simulink model "BoostConverterTestEnviroment"  (R2020a)
settings: Solver=ode15s  StartTime=0.0  StopTime=0.05  RelTol=1e-3
libraries: ee_lib x2, fl_lib x1, nesl_utility x1
settings Model: Creator=ykamatan  LastModifiedBy=ykamatan
settings SolverCC: MaxConsecutiveMinStep=10
settings DataIOCC: SaveOutput=off  SaveTime=off

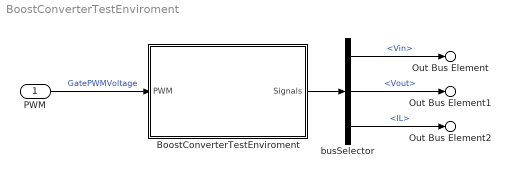
== system BoostConverterTestEnviroment ==
  PWM : Inport  OutDataTypeStr=double  PortDimensions=1  SampleTime=[2e-08,0]
  BoostConverterTestEnviroment : Subsystem  TreatAsAtomicUnit=on
  busSelector : BusSelector  OutputSignals=Vin,Vout,IL
  Out Bus Element : Outport  PortName=Signals  Element=Vin
  Out Bus Element1 : Outport  PortName=Signals  Element=Vout
  Out Bus Element2 : Outport  PortName=Signals  Element=IL
  wires:
  busSelector/3 -> Out Bus Element2/1  "<IL>"
  busSelector/2 -> Out Bus Element1/1  "<Vout>"
  busSelector/1 -> Out Bus Element/1  "<Vin>"
  BoostConverterTestEnviroment/1(Signals) -> busSelector/1
  PWM/1 -> BoostConverterTestEnviroment/1(PWM)  "GatePWMVoltage"

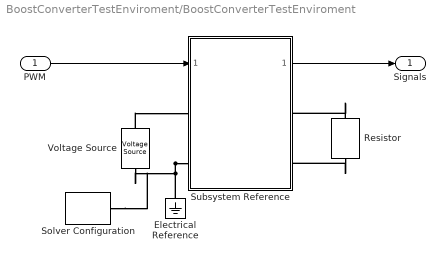
== system BoostConverterTestEnviroment/BoostConverterTestEnviroment ==
  PWM : Inport
  Electrical Reference : fl_lib/Electrical/Electrical Elements/Electrical Reference
  Resistor : ee_lib/Passive/Resistor  R=40 Ohm  R_tol=5  enable_R_tol=0  tol_distribution=1  nSigma=4  enable_operating_limits=0  operating_limit_action=2  max_working_voltage=100 V  power_rating=1 W  enable_faults=0  fault_action=1  R_faulted=inf Ohm  enable_temporal_fault=0  t_fault=1 s  enable_behavioral_fault=0  max_permissible_current=1 A  t_fail_on_current=1 s  noise_mode=0  sample_time=1e-3 s  repeatability=1  auto_seed=4144164703  user_seed=0  Tdevice=25 degC  alpha=3.93e-3 1/K  Tmeas=25 degC  thermal_mass=100 J/K  power_derating_T1=70 degC  power_derating_T2=155 degC  operating_temperature_range_vec=[-50, 150] degC  temperature_specify=off  temperature_priority=High  temperature=298.15 K  temperature_nominal_specify=off  temperature_nominal_unit=K  temperature_nominal_value=1
  Solver Configuration : nesl_utility/Solver Configuration  PhysicalDomain=network_engine_domain  SubClassName=solver  LeftPortType=input  RightPortType=generic  Tones=[]  Harmonics=[]  SimulateNoise=off  Profile=off  UseLocalSampling=off  EnableSwitchedLinearOptims=on  FrequencyDomain=off  UseCCode=off  RelTol=0.001  AbsTol=1e-06  MinStep=1e-09  ToWorkspace=off  RevertToSquareIcSolve=off  NumHomotopyIterations=100  PhasorMode=off  PhasorModeNumHarmonics=1  DoDC=off  ResidualTolerance=1e-09  UseLocalSolver=off  LocalSolverChoice=NE_BACKWARD_EULER_ADVANCER  LocalSolverSampleTime=0.001  DoFixedCost=off  MaxNonlinIter=3  MaxModeIter=2  LinearAlgebra=auto  EquationFormulation=NE_TIME_EF  DelaysMemoryBudget=1024  AutomaticFiltering=on  FilteringTimeConstant=0.001  PartitionStorageMethod=AS_NEEDED  PartitionMemoryBudget=1024  PartitionMethod=ROBUST
  Subsystem Reference : Subsystem  ReferencedSubsystem=BoostConverter
  Voltage Source : ee_lib/Sources/Voltage Source  dc_voltage=100 V  ac_voltage=0 V  ac_shift=0 rad  ac_frequency=60 Hz  noise_mode=0  PSD=0 V^2/Hz  repeatability=1  auto_seed=676943032  user_seed=0  sample_time=1e-3 s  i_specify=off  i_priority=None  i=0 A  i_nominal_specify=off  i_nominal_unit=A  i_nominal_value=1  v_specify=off  v_priority=None  v=0 V  v_nominal_specify=off  v_nominal_unit=V  v_nominal_value=1
  Signals : Outport
  wires:
  Subsystem Reference/1 -> Signals/1
  PWM/1 -> Subsystem Reference/1
  connections:
  Voltage Source/LConn1 -- Subsystem Reference/LConn1
  Resistor/RConn1 -- Subsystem Reference/RConn2
  Resistor/LConn1 -- Subsystem Reference/RConn1
  Subsystem Reference/LConn2 -- Electrical Reference/LConn1 -- Solver Configuration/RConn1 -- Voltage Source/RConn1
